simulink model "Control_test"  (R2014b)
settings: Solver=FixedStepDiscrete  StartTime=0.0  StopTime=Inf  FixedStep=0.001  RelTol=1e-3
PostLoadFcn:
  | , if any(exist('dsrtsu_mdlpostloadfcn', 'file') == [2, 3, 6]), try dsrtsu_mdlpostloadfcn('Execute', bdroot); catch fprintf('Error in PostLoadFcn (dsrtsu_mdlpostloadfcn) for model "%s":\n %s\n', bdroot, lasterr); end, end,
undefined symbols (not defined in the file or in its folder): dtLocal, slcm
libraries: rtican x163, simulink x14
(part 17 of 34)

== system Control_test/InputProcessing/RadarCanProcessing/Primary Target Selection ==
  IP : Inport
  Bus Creator : BusCreator
  Bus Selector : BusSelector  OutputSignals=ESR_Status4.CAN_TX_PATH_ID_ACC,Track01,Track02,Track03,Track04,Track05,Track06,Track07,Track08,Track09,Track10,Track11,Track12,Track13,Track14,Track15,Track16,Track17,Track18,Track19,Track20,Track21,Track22,Track23,Track24,Track25,Track26,Track27,Track28,Track29,Track30,Track31,Track32,Track33,Track34,Track35,Track36,Track37,Track38,Track39,Track40,Track41,Track42,Track43,Track44,Track45,Track46,Track47,Track48,Track49,Track50,Track51,Track52,Track53,Track54,Track55,Track56,Track57,Track58,Track59,Track60,Track61,Track62,Track63,Track64
  Default : Subsystem
  Demux : Demux  Outputs=12
  Multiport Switch1 : MultiPortSwitch  DataPortOrder=Zero-based contiguous  Inputs=65  zeroidx=on
  Terminator{,1..3,5..8} (8 alike) : Terminator
  PT : Outport
  wires:
  IP/1 -> Bus Selector/1
  Bus Selector/1 -> Multiport Switch1/1  "<CAN_TX_PATH_ID_ACC>"
  Bus Selector/2 -> Multiport Switch1/3  "<Track01>"
  Bus Selector/3 -> Multiport Switch1/4  "<Track02>"
  Bus Selector/4 -> Multiport Switch1/5  "<Track03>"
  Bus Selector/5 -> Multiport Switch1/6  "<Track04>"
  Bus Selector/6 -> Multiport Switch1/7  "<Track05>"
  Bus Selector/7 -> Multiport Switch1/8  "<Track06>"
  Bus Selector/8 -> Multiport Switch1/9  "<Track07>"
  Bus Selector/9 -> Multiport Switch1/10  "<Track08>"
  Bus Selector/10 -> Multiport Switch1/11  "<Track09>"
  Bus Selector/11 -> Multiport Switch1/12  "<Track10>"
  Bus Selector/12 -> Multiport Switch1/13  "<Track11>"
  Bus Selector/13 -> Multiport Switch1/14  "<Track12>"
  Bus Selector/14 -> Multiport Switch1/15  "<Track13>"
  Bus Selector/15 -> Multiport Switch1/16  "<Track14>"
  Bus Selector/16 -> Multiport Switch1/17  "<Track15>"
  Bus Selector/17 -> Multiport Switch1/18  "<Track16>"
  Bus Selector/18 -> Multiport Switch1/19  "<Track17>"
  Bus Selector/19 -> Multiport Switch1/20  "<Track18>"
  Bus Selector/20 -> Multiport Switch1/21  "<Track19>"
  Bus Selector/21 -> Multiport Switch1/22  "<Track20>"
  Bus Selector/22 -> Multiport Switch1/23  "<Track21>"
  Bus Selector/23 -> Multiport Switch1/24  "<Track22>"
  Bus Selector/24 -> Multiport Switch1/25  "<Track23>"
  Bus Selector/25 -> Multiport Switch1/26  "<Track24>"
  Bus Selector/26 -> Multiport Switch1/27  "<Track25>"
  Bus Selector/27 -> Multiport Switch1/28  "<Track26>"
  Bus Selector/28 -> Multiport Switch1/29  "<Track27>"
  Bus Selector/29 -> Multiport Switch1/30  "<Track28>"
  Bus Selector/30 -> Multiport Switch1/31  "<Track29>"
  Bus Selector/31 -> Multiport Switch1/32  "<Track30>"
  Bus Selector/32 -> Multiport Switch1/33  "<Track31>"
  Bus Selector/33 -> Multiport Switch1/34  "<Track32>"
  Bus Selector/34 -> Multiport Switch1/35  "<Track33>"
  Bus Selector/35 -> Multiport Switch1/36  "<Track34>"
  Bus Selector/36 -> Multiport Switch1/37  "<Track35>"
  Bus Selector/37 -> Multiport Switch1/38  "<Track36>"
  Bus Selector/38 -> Multiport Switch1/39  "<Track37>"
  Bus Selector/39 -> Multiport Switch1/40  "<Track38>"
  Bus Selector/40 -> Multiport Switch1/41  "<Track39>"
  Bus Selector/41 -> Multiport Switch1/42  "<Track40>"
  Bus Selector/42 -> Multiport Switch1/43  "<Track41>"
  Bus Selector/43 -> Multiport Switch1/44  "<Track42>"
  Bus Selector/44 -> Multiport Switch1/45  "<Track43>"
  Bus Selector/45 -> Multiport Switch1/46  "<Track44>"
  Bus Selector/46 -> Multiport Switch1/47  "<Track45>"
  Bus Selector/47 -> Multiport Switch1/48  "<Track46>"
  Bus Selector/48 -> Multiport Switch1/49  "<Track47>"
  Bus Selector/49 -> Multiport Switch1/50  "<Track48>"
  Bus Selector/50 -> Multiport Switch1/51  "<Track49>"
  Bus Selector/51 -> Multiport Switch1/52  "<Track50>"
  Bus Selector/52 -> Multiport Switch1/53  "<Track51>"
  Bus Selector/53 -> Multiport Switch1/54  "<Track52>"
  Bus Selector/54 -> Multiport Switch1/55  "<Track53>"
  Bus Selector/55 -> Multiport Switch1/56  "<Track54>"
  Bus Selector/56 -> Multiport Switch1/57  "<Track55>"
  Bus Selector/57 -> Multiport Switch1/58  "<Track56>"
  Bus Selector/58 -> Multiport Switch1/59  "<Track57>"
  Bus Selector/59 -> Multiport Switch1/60  "<Track58>"
  Bus Selector/60 -> Multiport Switch1/61  "<Track59>"
  Bus Selector/61 -> Multiport Switch1/62  "<Track60>"
  Bus Selector/62 -> Multiport Switch1/63  "<Track61>"
  Bus Selector/63 -> Multiport Switch1/64  "<Track62>"
  Bus Selector/64 -> Multiport Switch1/65  "<Track63>"
  Bus Selector/65 -> Multiport Switch1/66  "<Track64>"
  Default/1(Out1) -> Multiport Switch1/2
  Multiport Switch1/1 -> Demux/1
  Demux/1 -> Bus Creator/1  "RangeRate[m/s]"
  Demux/3 -> Bus Creator/2  "RangeAccel[m/s2]"
  Demux/7 -> Bus Creator/3  "Range[m]"
  Bus Creator/1 -> PT/1  "PT_Data"
  Demux/2 -> Terminator/1
  Demux/4 -> Terminator1/1
  Demux/5 -> Terminator2/1
  Demux/6 -> Terminator3/1
  Demux/9 -> Terminator5/1
  Demux/10 -> Terminator6/1
  Demux/11 -> Terminator7/1
  Demux/12 -> Terminator8/1
  Demux/8 -> Bus Creator/4  "Angle[deg]"

== system Control_test/InputProcessing/RadarCanProcessing/Status4 ==
  Bus Creator : BusCreator  Inputs=13
  Bus Selector : BusSelector  OutputSignals=CAN_TX_PATH_ID_ACC
  ESR_Status4 : rtican/RTICAN Receive (RX)   Reserved1=[]  Reserved2=[]  Reserved3=[]  Reserved4=[]  SfcnMessage=[]  Msg_Struct=[]  BoardTypeNo=[]  BoardNo=[]  ChannelNo=[]  Parameters=[]  DialogFcn=[]  UnitName=[]  Revision=[]  UnitValues=[]  DSProperties=struct('RTI',struct('Version',uint32(5),'BlockType',struct('isSLSource',uint8(1),'isSLSink',uint8(1),'isHWSource',uint8(0),'isHWSink',uint8(0),'isSetup',uint8(0),'isInline',uint8(1),'isNonInline',uint8(0),'isInterrupt',uint8(0),'isChannelwise',uint8(0)),'IOBoardType','RTICAN','UnitType','MESSAGE','Identifier','RX','DialogType','MSVC','BlockSet','RTICAN','SlaveProcessor','CAN'))  RTIBlockInterface=struct('OutputPortsWidth',int32([1 1 1 1 1 1 1 1 1 1 1 1 1]),'OutputPortsActive',[1 1 1 1 1 1 1 1 1 1 1 1 1],'OutputPortsName',{{'CAN_TX_PATH_ID_ACC_STAT','CAN_TX_AUTO_ALIGN_ANGLE','CAN_TX_PATH_ID_FCW_STAT','CAN_TX_PATH_ID_FCW_MOVE','CAN_TX_PATH_ID_CMBB_STAT','CAN_TX_PATH_ID_CMBB_MOVE','CAN_TX_PATH_ID_ACC','CAN_TX_ROLLING_COUNT_3','CAN_TX_MR_LR_MODE','CAN_TX_PARTIAL_BLOCKAGE','CAN_TX_SIDELOBE_BLOCKAGE','CAN_TX_LR_ONLY_GRATING_LOBE_DET','CAN_TX_TRUCK_TARGET_DET'}},'OutputPortsDataType',{{'SS_DOUBLE','SS_DOUBLE','SS_DOUBLE','SS_DOUBLE','SS_DOUBLE','SS_DOUBLE','SS_DOUBLE','SS_DOUBLE','SS_DOUBLE','SS_DOUBLE','SS_DOUBLE','SS_DOUBLE','SS_DOUBLE'}},'OutputPortsLabel',{{'CAN_TX_PATH_ID_ACC_STAT','CAN_TX_AUTO_ALIGN_ANGLE','CAN_TX_PATH_ID_FCW_STAT','CAN_TX_PATH_ID_FCW_MOVE','CAN_TX_PATH_ID_CMBB_STAT','CAN_TX_PATH_ID_CMBB_MOVE','CAN_TX_PATH_ID_ACC','CAN_TX_ROLLING_COUNT_3','CAN_TX_MR_LR_MODE','CAN_TX_PARTIAL_BLOCKAGE','CAN_TX_SIDELOBE_BLOCKAGE','CAN_TX_LR_ONLY_GRATING_LOBE_DET','CAN_TX_TRUCK_TARGET_DET'}},'OutputPortsLabelMode','ON','InputPortsWidth',int32(0),'InputPortsActive',0,'DialogFcn','rtican_message_interface_gui','BlockDisplay',{{'','center'}},'IconTransparency','on','ParameterTunableNames',{{}},'InitLevel',3,'BlockName',struct('Token',{{'ESR_Status4'}}),'SampleTime',{{0.01}},'TriggerPort',{{'none'}},'EnablePort',{{'none'}})  RTIBlockParameters=struct('BoardTypeNo',{{1,'OFF',[]}},'BoardNo',{{2,'ON',[1 16]}},'ChannelNo',{{2,'ON',[1 2]}},'Parameters',{{struct('DataFileSupport',struct('DataFileSelectedMaster',1,'DataFileSelectedLocal',0,'DataFileName','c:\users\mpc_car\documents\github\mpc-car\dbcfiles\esr_dv3_64tgt.dbc|','DataFileDate',{{{['26-Aug-2014 13:16:21']}}},'SelectedFile',['<no file selected>'],'InterfaceFcn','rtican_dbc_file_parser'),'Options',struct('StatusSelected',0,'TimeSelected',0,'DeltaTimeSelected',0,'BytePortSelected',0,'MessageLengthSelected',0,'TriggerPort',struct('Selected',0,'TriggerType',0),'UserCoding',struct('Selected',0,'InterfaceFile','UserDecodingFile','FcnName','UserDecodeFcn','InportSelected',0,'InportWidth',1,'OutportSelected',0,'OutportWidth',1),'EnablePortSelected',0,'SignalOnPortnameSelected',1,'UseRXService',0),'Message',struct('MsgOnBlocknameSelected',1,'MsgName','ESR_Status4','MsgIdFormat',0,'MsgId',1251,'MsgLength',8,'NumSignals',13,'SampleTime',0.01,'Signal',struct('SgnName',{'CAN_TX_PATH_ID_ACC_STAT','CAN_TX_AUTO_ALIGN_ANGLE','CAN_TX_PATH_ID_FCW_STAT','CAN_TX_PATH_ID_FCW_MOVE','CAN_TX_PATH_ID_CMBB_STAT','CAN_TX_PATH_ID_CMBB_MOVE','CAN_TX_PATH_ID_ACC','CAN_TX_ROLLING_COUNT_3','CAN_TX_MR_LR_MODE','CAN_TX_PARTIAL_BLOCKAGE','CAN_TX_SIDELOBE_BLOCKAGE','CAN_TX_LR_ONLY_GRATING_LOBE_DET','CAN_TX_TRUCK_TARGET_DET'},'SgnStartBit',{0,8,16,24,32,40,48,56,58,60,61,62,63},'SgnLength',{8,8,8,8,8,8,8,2,2,1,1,1,1},'SgnType',{0,0,0,0,0,0,0,0,0,0,0,0,0},'ModeValue',{-1,-1,-1,-1,-1,-1,-1,-1,-1,-1,-1,-1,-1},'DataType',{0,1,0,0,0,0,0,0,0,0,0,0,0},'ByteLayout',{2,2,2,2,2,2,2,2,2,2,2,2,2},'Factor',{1,0.0625,1,1,1,1,1,1,1,1,1,1,1},'Offset',{0,0,0,0,0,0,0,0,0,0,0,0,0},'SgnComment',{{''},{''},{''},{''},{''},{''},{''},{''},{''},{''},{''},{''},{''}},'SgnUnit',{'','','','','','','','','','','','',''},'Min',{0,-8,0,0,0,0,0,0,0,0,0,0,0},'Max',{0,7.9375,0,0,0,0,0,0,3,0,0,0,0},'SLDataType',{'SS_DOUBLE','SS_DOUBLE','SS_DOUBLE','SS_DOUBLE','SS_DOUBLE','SS_DOUBLE','SS_DOUBLE','SS_DOUBLE','SS_DOUBLE','SS_DOUBLE','SS_DOUBLE','SS_DOUBLE','SS_DOUBLE'}),'MsgIdNumFormat',0,'MsgComment',{{''}}),'Version',1.2,'general',struct('isFromLib',0)),'OFF',[]}},'GroupId',{{struct('Group',{{'RTICAN'}},'No',4,'Behavior',{{'NAMECHANGE'}},'BlockType',{{'SINK'}},'NameChangeFlag',0),'OFF',[]}},'SFcnRTICANMessage',{{struct('MsgType','RX','SFcnPortType','Scalar','MsgName','ESR_Status4','MsgIdFormat','STD','MsgId',1251,'MsgLength',8,'NumSignals',13,'SampleTime',0.01,'Signal',struct('SgnName',{'CAN_TX_PATH_ID_ACC_STAT','CAN_TX_AUTO_ALIGN_ANGLE','CAN_TX_PATH_ID_FCW_STAT','CAN_TX_PATH_ID_FCW_MOVE','CAN_TX_PATH_ID_CMBB_STAT','CAN_TX_PATH_ID_CMBB_MOVE','CAN_TX_PATH_ID_ACC','CAN_TX_ROLLING_COUNT_3','CAN_TX_MR_LR_MODE','CAN_TX_PARTIAL_BLOCKAGE','CAN_TX_SIDELOBE_BLOCKAGE','CAN_TX_LR_ONLY_GRATING_LOBE_DET','CAN_TX_TRUCK_TARGET_DET'},'SgnStartBit',{0,8,16,24,32,40,48,56,58,60,61,62,63},'SgnLength',{8,8,8,8,8,8,8,2,2,1,1,1,1},'SgnType',{'standard','standard','standard','standard','standard','standard','standard','standard','standard','standard','standard','standard','standard'},'ModeValue',{-1,-1,-1,-1,-1,-1,-1,-1,-1,-1,-1,-1,-1},'DataType',{['unsigned int'],['signed int'],['unsigned int'],['unsigned int'],['unsigned int'],['unsigned int'],['unsigned int'],['unsigned int'],['unsigned int'],['unsigned int'],['unsigned int'],['unsigned int'],['unsigned int']},'ByteLayout',{['motorola back.'],['motorola back.'],['motorola back.'],['motorola back.'],['motorola back.'],['motorola back.'],['motorola back.'],['motorola back.'],['motorola back.'],['motorola back.'],['motorola back.'],['motorola back.'],['motorola back.']},'Factor',{1,0.0625,1,1,1,1,1,1,1,1,1,1,1},'Offset',{0,0,0,0,0,0,0,0,0,0,0,0,0},'SLDataType',{'SS_DOUBLE','SS_DOUBLE','SS_DOUBLE','SS_DOUBLE','SS_DOUBLE','SS_DOUBLE','SS_DOUBLE','SS_DOUBLE','SS_DOUBLE','SS_DOUBLE','SS_DOUBLE','SS_DOUBLE','SS_DOUBLE'}),'StatusSelected','no','TimeSelected','no','DeltaTimeSelected','no','BytePortSelected','no','MessageLengthSelected','no','TriggerPort',struct('Selected','no','TriggerType',0),'UserCoding',struct('Selected','no','InterfaceFile','UserDecodingFile','FcnName','UserDecodeFcn','InportSelected','no','InportWidth',1,'OutportSelected','no','OutportWidth',1),'EnablePortSelected','no','UseRXService','no','BoardType','DS1','BoardNo',2,'ControllerNo',2),'OFF',[]}},'TLCFileName',{{'rtican_rx_message','OFF',[]}})  RTISFcnParameters=struct('SFcnRTICANMessage','struct','TLCFileName','char')  RTIBlockParaDefault=struct('BoardTypeNo',4302,'BoardNo',1,'ChannelNo',1,'Parameters',struct('DataFileSupport',struct('DataFileSelectedMaster',0,'DataFileSelectedLocal',0,'DataFileName','','DataFileDate','','SelectedFile',['<no file selected>']),'Options',struct('StatusSelected',1,'TimeSelected',1,'DeltaTimeSelected',1,'BytePortSelected',0,'MessageLengthSelected',0,'TriggerPort',struct('Selected',0,'TriggerType','rising'),'UserCoding',struct('Selected',0,'InterfaceFile','UserDecodingFile','FcnName','UserDecodeFcn','InportSelected',0,'InportWidth',1,'OutportSelected',0,'OutportWidth',1),'EnablePortSelected',0,'SignalOnPortnameSelected',1,'UseRXService',0),'Message',struct('MsgOnBlocknameSelected',0,'MsgName',['RX Message'],'MsgIdFormat',0,'MsgId',100,'MsgLength',8,'NumSignals',1,'SampleTime',-1,'Signal',struct('SgnName',['RX signal'],'SgnStartBit',0,'SgnLength',8,'SgnType',0,'ModeValue',-1,'DataType',0,'SLDataType','SS_DOUBLE','ByteLayout',0,'Factor',1,'Offset',0,'Min',0,'Max',255,'SgnComment',{{}},'SgnUnit',''),'MsgIdNumFormat',0,'MsgComment',{{''}}),'Version',1.2,'general',struct('isFromLib',1)),'GroupId',struct('Group',{{'RTICAN'}},'No',1,'Behavior',{{'NAMECHANGE'}},'BlockType',{{'SINK'}},'NameChangeFlag',0),'SFcnRTICANMessage',struct('MsgType','RX','MsgName',['RX Message'],'MsgIdFormat','STD','MsgId',100,'MsgLength',8,'NumSignals',1,'SampleTime',-1,'Signal',struct('SgnName',['RX signal'],'SgnStartBit',0,'SgnLength',8,'SgnType','standard','ModeValue',-1,'DataType',['unsigned int'],'ByteLayout',['little endian'],'SLDataType','SS_DOUBLE','Factor',1,'Offset',0),'StatusSelected','yes','TimeSelected','yes','DeltaTimeSelected','yes','BytePortSelected','no','MessageLengthSelected','no','EnablePortSelected','no','UserCoding',struct('Selected','no','InterfaceFile','UserDecodingFile','FcnName','UserDecodeFcn','InportSelected','no','InportWidth',1,'OutportSelected','no','OutportWidth',1),'TriggerPort',struct('Selected','no','TriggerType','rising'),'UseRXService','no','BoardType','DS4302','BoardNo',1,'ControllerNo',1,'SFcnPortType','Scalar'),'TLCFileName','rtican_rx_message')
      settings: AttributesFormatString=Group Id: RTICAN4\n
  CAN_TX_PATH_ID_ACC : Outport
  wires:
  ESR_Status4/1 -> Bus Creator/1  "CAN_TX_PATH_ID_ACC_STAT"
  ESR_Status4/2 -> Bus Creator/2  "CAN_TX_AUTO_ALIGN_ANGLE"
  ESR_Status4/3 -> Bus Creator/3  "CAN_TX_PATH_ID_FCW_STAT"
  ESR_Status4/4 -> Bus Creator/4  "CAN_TX_PATH_ID_FCW_MOVE"
  ESR_Status4/5 -> Bus Creator/5  "CAN_TX_PATH_ID_CMBB_STAT"
  ESR_Status4/6 -> Bus Creator/6  "CAN_TX_PATH_ID_CMBB_MOVE"
  ESR_Status4/7 -> Bus Creator/7  "CAN_TX_PATH_ID_ACC"
  ESR_Status4/8 -> Bus Creator/8  "CAN_TX_ROLLING_COUNT_3"
  ESR_Status4/9 -> Bus Creator/9  "CAN_TX_MR_LR_MODE"
  ESR_Status4/10 -> Bus Creator/10  "CAN_TX_PARTIAL_BLOCKAGE"
  ESR_Status4/11 -> Bus Creator/11  "CAN_TX_SIDELOBE_BLOCKAGE"
  ESR_Status4/12 -> Bus Creator/12  "CAN_TX_LR_ONLY_GRATING_LOBE_DET"
  ESR_Status4/13 -> Bus Creator/13  "CAN_TX_TRUCK_TARGET_DET"
  Bus Creator/1 -> Bus Selector/1  "Status4"
  Bus Selector/1 -> CAN_TX_PATH_ID_ACC/1  "<CAN_TX_PATH_ID_ACC>"

== system Control_test/InputProcessing/RadarCanProcessing/Track01 ==
  Bus Creator : BusCreator  Inputs=12
  ESR_Track01 : rtican/RTICAN Receive (RX)   Reserved1=[]  Reserved2=[]  Reserved3=[]  Reserved4=[]  SfcnMessage=[]  Msg_Struct=[]  BoardTypeNo=[]  BoardNo=[]  ChannelNo=[]  Parameters=[]  DialogFcn=[]  UnitName=[]  Revision=[]  UnitValues=[]  DSProperties=struct('RTI',struct('Version',uint32(5),'BlockType',struct('isSLSource',uint8(1),'isSLSink',uint8(1),'isHWSource',uint8(0),'isHWSink',uint8(0),'isSetup',uint8(0),'isInline',uint8(1),'isNonInline',uint8(0),'isInterrupt',uint8(0),'isChannelwise',uint8(0)),'IOBoardType','RTICAN','UnitType','MESSAGE','Identifier','RX','DialogType','MSVC','BlockSet','RTICAN','SlaveProcessor','CAN'))  RTIBlockInterface=struct('OutputPortsWidth',int32([1 1 1 1 1 1 1 1 1 1 1 1]),'OutputPortsActive',[1 1 1 1 1 1 1 1 1 1 1 1],'OutputPortsName',{{'CAN_TX_TRACK_RANGE_RATE_01','CAN_TX_TRACK_MED_RANGE_MODE_01','CAN_TX_TRACK_RANGE_ACCEL_01','CAN_TX_TRACK_WIDTH_01','CAN_TX_TRACK_ROLLING_COUNT_01','CAN_TX_TRACK_BRIDGE_OBJECT_01','CAN_TX_TRACK_RANGE_01','CAN_TX_TRACK_ANGLE_01','CAN_TX_TRACK_STATUS_01','CAN_TX_TRACK_ONCOMING_01','CAN_TX_TRACK_GROUPING_CHANGED_01','CAN_TX_TRACK_LAT_RATE_01'}},'OutputPortsDataType',{{'SS_DOUBLE','SS_DOUBLE','SS_DOUBLE','SS_DOUBLE','SS_DOUBLE','SS_DOUBLE','SS_DOUBLE','SS_DOUBLE','SS_DOUBLE','SS_DOUBLE','SS_DOUBLE','SS_DOUBLE'}},'OutputPortsLabel',{{'CAN_TX_TRACK_RANGE_RATE_01','CAN_TX_TRACK_MED_RANGE_MODE_01','CAN_TX_TRACK_RANGE_ACCEL_01','CAN_TX_TRACK_WIDTH_01','CAN_TX_TRACK_ROLLING_COUNT_01','CAN_TX_TRACK_BRIDGE_OBJECT_01','CAN_TX_TRACK_RANGE_01','CAN_TX_TRACK_ANGLE_01','CAN_TX_TRACK_STATUS_01','CAN_TX_TRACK_ONCOMING_01','CAN_TX_TRACK_GROUPING_CHANGED_01','CAN_TX_TRACK_LAT_RATE_01'}},'OutputPortsLabelMode','ON','InputPortsWidth',int32(0),'InputPortsActive',0,'DialogFcn','rtican_message_interface_gui','BlockDisplay',{{'','center'}},'IconTransparency','on','ParameterTunableNames',{{}},'InitLevel',3,'BlockName',struct('Token',{{'ESR_Track01'}}),'SampleTime',{{0.01}},'TriggerPort',{{'none'}},'EnablePort',{{'none'}})  RTIBlockParameters=struct('BoardTypeNo',{{1,'OFF',[]}},'BoardNo',{{2,'ON',[1 16]}},'ChannelNo',{{2,'ON',[1 2]}},'Parameters',{{struct('DataFileSupport',struct('DataFileSelectedMaster',1,'DataFileSelectedLocal',1,'DataFileName','c:\users\mpc_car\documents\github\mpc-car\controller\dbcfiles\esr_dv3_64tgt.dbc|','DataFileDate',['26-Aug-2014 13:16:21'],'SelectedFile','..\..\dbcfiles\esr_dv3_64tgt.dbc','InterfaceFcn','rtican_dbc_file_parser'),'Options',struct('StatusSelected',0,'TimeSelected',0,'DeltaTimeSelected',0,'BytePortSelected',0,'MessageLengthSelected',0,'TriggerPort',struct('Selected',0,'TriggerType',0),'UserCoding',struct('Selected',0,'InterfaceFile','UserDecodingFile','FcnName','UserDecodeFcn','InportSelected',0,'InportWidth',1,'OutportSelected',0,'OutportWidth',1),'EnablePortSelected',0,'SignalOnPortnameSelected',1,'UseRXService',0),'Message',struct('MsgOnBlocknameSelected',1,'MsgName','ESR_Track01','MsgIdFormat',0,'MsgId',1280,'MsgLength',8,'NumSignals',12,'SampleTime',0.01,'Signal',struct('SgnName',{'CAN_TX_TRACK_RANGE_RATE_01','CAN_TX_TRACK_MED_RANGE_MODE_01','CAN_TX_TRACK_RANGE_ACCEL_01','CAN_TX_TRACK_WIDTH_01','CAN_TX_TRACK_ROLLING_COUNT_01','CAN_TX_TRACK_BRIDGE_OBJECT_01','CAN_TX_TRACK_RANGE_01','CAN_TX_TRACK_ANGLE_01','CAN_TX_TRACK_STATUS_01','CAN_TX_TRACK_ONCOMING_01','CAN_TX_TRACK_GROUPING_CHANGED_01','CAN_TX_TRACK_LAT_RATE_01'},'SgnStartBit',{0,14,16,26,30,31,32,43,53,56,57,58},'SgnLength',{14,2,10,4,1,1,11,10,3,1,1,6},'ByteLayout',{2,2,2,2,2,2,2,2,2,2,2,2},'Factor',{0.01,1,0.05,0.5,1,1,0.1,0.1,1,1,1,0.25},'Offset',{0,0,0,0,0,0,0,0,0,0,0,0},'SgnComment',{'','','','','','','','','','','',''},'SgnUnit',{'m/s','','m/s/s','m','','','m','deg','','','',''},'Min',{-81.92,0,-25.6,0,0,0,0,-51.2,0,0,0,-8},'Max',{81.91,3,25.55,7.5,1,0,204.7,51.1,7,0,0,7.75},'SgnType',{0,0,0,0,0,0,0,0,0,0,0,0},'SLDataType',{'SS_DOUBLE','SS_DOUBLE','SS_DOUBLE','SS_DOUBLE','SS_DOUBLE','SS_DOUBLE','SS_DOUBLE','SS_DOUBLE','SS_DOUBLE','SS_DOUBLE','SS_DOUBLE','SS_DOUBLE'},'DataType',{1,0,1,0,0,0,0,1,0,0,0,1},'ModeValue',{-1,-1,-1,-1,-1,-1,-1,-1,-1,-1,-1,-1}),'MsgIdNumFormat',0,'MsgComment',{{''}}),'Version',1.2,'general',struct('isFromLib',0)),'OFF',[]}},'GroupId',{{struct('Group',{{'RTICAN'}},'No',4,'Behavior',{{'NAMECHANGE'}},'BlockType',{{'SINK'}},'NameChangeFlag',0),'OFF',[]}},'SFcnRTICANMessage',{{struct('MsgType','RX','SFcnPortType','Scalar','MsgName','ESR_Track01','MsgIdFormat','STD','MsgId',1280,'MsgLength',8,'NumSignals',12,'SampleTime',0.01,'Signal',struct('SgnName',{'CAN_TX_TRACK_RANGE_RATE_01','CAN_TX_TRACK_MED_RANGE_MODE_01','CAN_TX_TRACK_RANGE_ACCEL_01','CAN_TX_TRACK_WIDTH_01','CAN_TX_TRACK_ROLLING_COUNT_01','CAN_TX_TRACK_BRIDGE_OBJECT_01','CAN_TX_TRACK_RANGE_01','CAN_TX_TRACK_ANGLE_01','CAN_TX_TRACK_STATUS_01','CAN_TX_TRACK_ONCOMING_01','CAN_TX_TRACK_GROUPING_CHANGED_01','CAN_TX_TRACK_LAT_RATE_01'},'SgnStartBit',{0,14,16,26,30,31,32,43,53,56,57,58},'SgnLength',{14,2,10,4,1,1,11,10,3,1,1,6},'ByteLayout',{['motorola back.'],['motorola back.'],['motorola back.'],['motorola back.'],['motorola back.'],['motorola back.'],['motorola back.'],['motorola back.'],['motorola back.'],['motorola back.'],['motorola back.'],['motorola back.']},'Factor',{0.01,1,0.05,0.5,1,1,0.1,0.1,1,1,1,0.25},'Offset',{0,0,0,0,0,0,0,0,0,0,0,0},'SgnType',{'standard','standard','standard','standard','standard','standard','standard','standard','standard','standard','standard','standard'},'SLDataType',{'SS_DOUBLE','SS_DOUBLE','SS_DOUBLE','SS_DOUBLE','SS_DOUBLE','SS_DOUBLE','SS_DOUBLE','SS_DOUBLE','SS_DOUBLE','SS_DOUBLE','SS_DOUBLE','SS_DOUBLE'},'DataType',{['signed int'],['unsigned int'],['signed int'],['unsigned int'],['unsigned int'],['unsigned int'],['unsigned int'],['signed int'],['unsigned int'],['unsigned int'],['unsigned int'],['signed int']},'ModeValue',{-1,-1,-1,-1,-1,-1,-1,-1,-1,-1,-1,-1}),'StatusSelected','no','TimeSelected','no','DeltaTimeSelected','no','BytePortSelected','no','MessageLengthSelected','no','TriggerPort',struct('Selected','no','TriggerType',0),'UserCoding',struct('Selected','no','InterfaceFile','UserDecodingFile','FcnName','UserDecodeFcn','InportSelected','no','InportWidth',1,'OutportSelected','no','OutportWidth',1),'EnablePortSelected','no','UseRXService','no','BoardType','DS1','BoardNo',2,'ControllerNo',2),'OFF',[]}},'TLCFileName',{{'rtican_rx_message','OFF',[]}})  RTISFcnParameters=struct('SFcnRTICANMessage','struct','TLCFileName','char')  RTIBlockParaDefault=struct('BoardTypeNo',4302,'BoardNo',1,'ChannelNo',1,'Parameters',struct('DataFileSupport',struct('DataFileSelectedMaster',0,'DataFileSelectedLocal',0,'DataFileName','','DataFileDate','','SelectedFile',['<no file selected>']),'Options',struct('StatusSelected',1,'TimeSelected',1,'DeltaTimeSelected',1,'BytePortSelected',0,'MessageLengthSelected',0,'TriggerPort',struct('Selected',0,'TriggerType','rising'),'UserCoding',struct('Selected',0,'InterfaceFile','UserDecodingFile','FcnName','UserDecodeFcn','InportSelected',0,'InportWidth',1,'OutportSelected',0,'OutportWidth',1),'EnablePortSelected',0,'SignalOnPortnameSelected',1,'UseRXService',0),'Message',struct('MsgOnBlocknameSelected',0,'MsgName',['RX Message'],'MsgIdFormat',0,'MsgId',100,'MsgLength',8,'NumSignals',1,'SampleTime',-1,'Signal',struct('SgnName',['RX signal'],'SgnStartBit',0,'SgnLength',8,'SgnType',0,'ModeValue',-1,'DataType',0,'SLDataType','SS_DOUBLE','ByteLayout',0,'Factor',1,'Offset',0,'Min',0,'Max',255,'SgnComment',{{}},'SgnUnit',''),'MsgIdNumFormat',0,'MsgComment',{{''}}),'Version',1.2,'general',struct('isFromLib',1)),'GroupId',struct('Group',{{'RTICAN'}},'No',1,'Behavior',{{'NAMECHANGE'}},'BlockType',{{'SINK'}},'NameChangeFlag',0),'SFcnRTICANMessage',struct('MsgType','RX','MsgName',['RX Message'],'MsgIdFormat','STD','MsgId',100,'MsgLength',8,'NumSignals',1,'SampleTime',-1,'Signal',struct('SgnName',['RX signal'],'SgnStartBit',0,'SgnLength',8,'SgnType','standard','ModeValue',-1,'DataType',['unsigned int'],'ByteLayout',['little endian'],'SLDataType','SS_DOUBLE','Factor',1,'Offset',0),'StatusSelected','yes','TimeSelected','yes','DeltaTimeSelected','yes','BytePortSelected','no','MessageLengthSelected','no','EnablePortSelected','no','UserCoding',struct('Selected','no','InterfaceFile','UserDecodingFile','FcnName','UserDecodeFcn','InportSelected','no','InportWidth',1,'OutportSelected','no','OutportWidth',1),'TriggerPort',struct('Selected','no','TriggerType','rising'),'UseRXService','no','BoardType','DS4302','BoardNo',1,'ControllerNo',1,'SFcnPortType','Scalar'),'TLCFileName','rtican_rx_message')
      settings: AttributesFormatString=Group Id: RTICAN4\n
  Out1 : Outport
  wires:
  ESR_Track01/1 -> Bus Creator/1  "CAN_TX_TRACK_RANGE_RATE_01"
  ESR_Track01/2 -> Bus Creator/2  "CAN_TX_TRACK_MED_RANGE_MODE_01"
  ESR_Track01/3 -> Bus Creator/3  "CAN_TX_TRACK_RANGE_ACCEL_01"
  ESR_Track01/4 -> Bus Creator/4  "CAN_TX_TRACK_WIDTH_01"
  ESR_Track01/5 -> Bus Creator/5  "CAN_TX_TRACK_ROLLING_COUNT_01"
  ESR_Track01/6 -> Bus Creator/6  "CAN_TX_TRACK_BRIDGE_OBJECT_01"
  ESR_Track01/7 -> Bus Creator/7  "CAN_TX_TRACK_RANGE_01"
  ESR_Track01/8 -> Bus Creator/8  "CAN_TX_TRACK_ANGLE_01"
  ESR_Track01/9 -> Bus Creator/9  "CAN_TX_TRACK_STATUS_01"
  ESR_Track01/10 -> Bus Creator/10  "CAN_TX_TRACK_ONCOMING_01"
  ESR_Track01/11 -> Bus Creator/11  "CAN_TX_TRACK_GROUPING_CHANGED_01"
  ESR_Track01/12 -> Bus Creator/12  "CAN_TX_TRACK_LAT_RATE_01"
  Bus Creator/1 -> Out1/1  "Track01"

== system Control_test/InputProcessing/RadarCanProcessing/Track02 ==
  Bus Creator : BusCreator  Inputs=12
  ESR_Track02 : rtican/RTICAN Receive (RX)   Reserved1=[]  Reserved2=[]  Reserved3=[]  Reserved4=[]  SfcnMessage=[]  Msg_Struct=[]  BoardTypeNo=[]  BoardNo=[]  ChannelNo=[]  Parameters=[]  DialogFcn=[]  UnitName=[]  Revision=[]  UnitValues=[]  DSProperties=struct('RTI',struct('Version',uint32(5),'BlockType',struct('isSLSource',uint8(1),'isSLSink',uint8(1),'isHWSource',uint8(0),'isHWSink',uint8(0),'isSetup',uint8(0),'isInline',uint8(1),'isNonInline',uint8(0),'isInterrupt',uint8(0),'isChannelwise',uint8(0)),'IOBoardType','RTICAN','UnitType','MESSAGE','Identifier','RX','DialogType','MSVC','BlockSet','RTICAN','SlaveProcessor','CAN'))  RTIBlockInterface=struct('OutputPortsWidth',int32([1 1 1 1 1 1 1 1 1 1 1 1]),'OutputPortsActive',[1 1 1 1 1 1 1 1 1 1 1 1],'OutputPortsName',{{'CAN_TX_TRACK_RANGE_RATE_02','CAN_TX_TRACK_MED_RANGE_MODE_02','CAN_TX_TRACK_RANGE_ACCEL_02','CAN_TX_TRACK_WIDTH_02','CAN_TX_TRACK_ROLLING_COUNT_02','CAN_TX_TRACK_BRIDGE_OBJECT_02','CAN_TX_TRACK_RANGE_02','CAN_TX_TRACK_ANGLE_02','CAN_TX_TRACK_STATUS_02','CAN_TX_TRACK_ONCOMING_02','CAN_TX_TRACK_GROUPING_CHANGED_02','CAN_TX_TRACK_LAT_RATE_02'}},'OutputPortsDataType',{{'SS_DOUBLE','SS_DOUBLE','SS_DOUBLE','SS_DOUBLE','SS_DOUBLE','SS_DOUBLE','SS_DOUBLE','SS_DOUBLE','SS_DOUBLE','SS_DOUBLE','SS_DOUBLE','SS_DOUBLE'}},'OutputPortsLabel',{{'CAN_TX_TRACK_RANGE_RATE_02','CAN_TX_TRACK_MED_RANGE_MODE_02','CAN_TX_TRACK_RANGE_ACCEL_02','CAN_TX_TRACK_WIDTH_02','CAN_TX_TRACK_ROLLING_COUNT_02','CAN_TX_TRACK_BRIDGE_OBJECT_02','CAN_TX_TRACK_RANGE_02','CAN_TX_TRACK_ANGLE_02','CAN_TX_TRACK_STATUS_02','CAN_TX_TRACK_ONCOMING_02','CAN_TX_TRACK_GROUPING_CHANGED_02','CAN_TX_TRACK_LAT_RATE_02'}},'OutputPortsLabelMode','ON','InputPortsWidth',int32(0),'InputPortsActive',0,'DialogFcn','rtican_message_interface_gui','BlockDisplay',{{'','center'}},'IconTransparency','on','ParameterTunableNames',{{}},'InitLevel',3,'BlockName',struct('Token',{{'ESR_Track02'}}),'SampleTime',{{0.01}},'TriggerPort',{{'none'}},'EnablePort',{{'none'}})  RTIBlockParameters=struct('BoardTypeNo',{{1,'OFF',[]}},'BoardNo',{{2,'ON',[1 16]}},'ChannelNo',{{2,'ON',[1 2]}},'Parameters',{{struct('DataFileSupport',struct('DataFileSelectedMaster',1,'DataFileSelectedLocal',1,'DataFileName','c:\users\mpc_car\documents\github\mpc-car\controller\dbcfiles\esr_dv3_64tgt.dbc|','DataFileDate',['26-Aug-2014 13:16:21'],'SelectedFile','..\..\dbcfiles\esr_dv3_64tgt.dbc','InterfaceFcn','rtican_dbc_file_parser'),'Options',struct('StatusSelected',0,'TimeSelected',0,'DeltaTimeSelected',0,'BytePortSelected',0,'MessageLengthSelected',0,'TriggerPort',struct('Selected',0,'TriggerType',0),'UserCoding',struct('Selected',0,'InterfaceFile','UserDecodingFile','FcnName','UserDecodeFcn','InportSelected',0,'InportWidth',1,'OutportSelected',0,'OutportWidth',1),'EnablePortSelected',0,'SignalOnPortnameSelected',1,'UseRXService',0),'Message',struct('MsgOnBlocknameSelected',1,'MsgName','ESR_Track02','MsgIdFormat',0,'MsgId',1281,'MsgLength',8,'NumSignals',12,'SampleTime',0.01,'Signal',struct('SgnName',{'CAN_TX_TRACK_RANGE_RATE_02','CAN_TX_TRACK_MED_RANGE_MODE_02','CAN_TX_TRACK_RANGE_ACCEL_02','CAN_TX_TRACK_WIDTH_02','CAN_TX_TRACK_ROLLING_COUNT_02','CAN_TX_TRACK_BRIDGE_OBJECT_02','CAN_TX_TRACK_RANGE_02','CAN_TX_TRACK_ANGLE_02','CAN_TX_TRACK_STATUS_02','CAN_TX_TRACK_ONCOMING_02','CAN_TX_TRACK_GROUPING_CHANGED_02','CAN_TX_TRACK_LAT_RATE_02'},'SgnStartBit',{0,14,16,26,30,31,32,43,53,56,57,58},'SgnLength',{14,2,10,4,1,1,11,10,3,1,1,6},'ByteLayout',{2,2,2,2,2,2,2,2,2,2,2,2},'Factor',{0.01,1,0.05,0.5,1,1,0.1,0.1,1,1,1,0.25},'Offset',{0,0,0,0,0,0,0,0,0,0,0,0},'SgnComment',{'','','','','','','','','','','',''},'SgnUnit',{'m/s','','m/s/s','m','','','m','deg','','','',''},'Min',{-81.92,0,-25.6,0,0,0,0,-51.2,0,0,0,-8},'Max',{81.91,3,25.55,7.5,1,0,204.7,51.1,7,0,0,7.75},'SgnType',{0,0,0,0,0,0,0,0,0,0,0,0},'SLDataType',{'SS_DOUBLE','SS_DOUBLE','SS_DOUBLE','SS_DOUBLE','SS_DOUBLE','SS_DOUBLE','SS_DOUBLE','SS_DOUBLE','SS_DOUBLE','SS_DOUBLE','SS_DOUBLE','SS_DOUBLE'},'DataType',{1,0,1,0,0,0,0,1,0,0,0,1},'ModeValue',{-1,-1,-1,-1,-1,-1,-1,-1,-1,-1,-1,-1}),'MsgIdNumFormat',0,'MsgComment',{{''}}),'Version',1.2,'general',struct('isFromLib',0)),'OFF',[]}},'GroupId',{{struct('Group',{{'RTICAN'}},'No',4,'Behavior',{{'NAMECHANGE'}},'BlockType',{{'SINK'}},'NameChangeFlag',0),'OFF',[]}},'SFcnRTICANMessage',{{struct('MsgType','RX','SFcnPortType','Scalar','MsgName','ESR_Track02','MsgIdFormat','STD','MsgId',1281,'MsgLength',8,'NumSignals',12,'SampleTime',0.01,'Signal',struct('SgnName',{'CAN_TX_TRACK_RANGE_RATE_02','CAN_TX_TRACK_MED_RANGE_MODE_02','CAN_TX_TRACK_RANGE_ACCEL_02','CAN_TX_TRACK_WIDTH_02','CAN_TX_TRACK_ROLLING_COUNT_02','CAN_TX_TRACK_BRIDGE_OBJECT_02','CAN_TX_TRACK_RANGE_02','CAN_TX_TRACK_ANGLE_02','CAN_TX_TRACK_STATUS_02','CAN_TX_TRACK_ONCOMING_02','CAN_TX_TRACK_GROUPING_CHANGED_02','CAN_TX_TRACK_LAT_RATE_02'},'SgnStartBit',{0,14,16,26,30,31,32,43,53,56,57,58},'SgnLength',{14,2,10,4,1,1,11,10,3,1,1,6},'ByteLayout',{['motorola back.'],['motorola back.'],['motorola back.'],['motorola back.'],['motorola back.'],['motorola back.'],['motorola back.'],['motorola back.'],['motorola back.'],['motorola back.'],['motorola back.'],['motorola back.']},'Factor',{0.01,1,0.05,0.5,1,1,0.1,0.1,1,1,1,0.25},'Offset',{0,0,0,0,0,0,0,0,0,0,0,0},'SgnType',{'standard','standard','standard','standard','standard','standard','standard','standard','standard','standard','standard','standard'},'SLDataType',{'SS_DOUBLE','SS_DOUBLE','SS_DOUBLE','SS_DOUBLE','SS_DOUBLE','SS_DOUBLE','SS_DOUBLE','SS_DOUBLE','SS_DOUBLE','SS_DOUBLE','SS_DOUBLE','SS_DOUBLE'},'DataType',{['signed int'],['unsigned int'],['signed int'],['unsigned int'],['unsigned int'],['unsigned int'],['unsigned int'],['signed int'],['unsigned int'],['unsigned int'],['unsigned int'],['signed int']},'ModeValue',{-1,-1,-1,-1,-1,-1,-1,-1,-1,-1,-1,-1}),'StatusSelected','no','TimeSelected','no','DeltaTimeSelected','no','BytePortSelected','no','MessageLengthSelected','no','TriggerPort',struct('Selected','no','TriggerType',0),'UserCoding',struct('Selected','no','InterfaceFile','UserDecodingFile','FcnName','UserDecodeFcn','InportSelected','no','InportWidth',1,'OutportSelected','no','OutportWidth',1),'EnablePortSelected','no','UseRXService','no','BoardType','DS1','BoardNo',2,'ControllerNo',2),'OFF',[]}},'TLCFileName',{{'rtican_rx_message','OFF',[]}})  RTISFcnParameters=struct('SFcnRTICANMessage','struct','TLCFileName','char')  RTIBlockParaDefault=struct('BoardTypeNo',4302,'BoardNo',1,'ChannelNo',1,'Parameters',struct('DataFileSupport',struct('DataFileSelectedMaster',0,'DataFileSelectedLocal',0,'DataFileName','','DataFileDate','','SelectedFile',['<no file selected>']),'Options',struct('StatusSelected',1,'TimeSelected',1,'DeltaTimeSelected',1,'BytePortSelected',0,'MessageLengthSelected',0,'TriggerPort',struct('Selected',0,'TriggerType','rising'),'UserCoding',struct('Selected',0,'InterfaceFile','UserDecodingFile','FcnName','UserDecodeFcn','InportSelected',0,'InportWidth',1,'OutportSelected',0,'OutportWidth',1),'EnablePortSelected',0,'SignalOnPortnameSelected',1,'UseRXService',0),'Message',struct('MsgOnBlocknameSelected',0,'MsgName',['RX Message'],'MsgIdFormat',0,'MsgId',100,'MsgLength',8,'NumSignals',1,'SampleTime',-1,'Signal',struct('SgnName',['RX signal'],'SgnStartBit',0,'SgnLength',8,'SgnType',0,'ModeValue',-1,'DataType',0,'SLDataType','SS_DOUBLE','ByteLayout',0,'Factor',1,'Offset',0,'Min',0,'Max',255,'SgnComment',{{}},'SgnUnit',''),'MsgIdNumFormat',0,'MsgComment',{{''}}),'Version',1.2,'general',struct('isFromLib',1)),'GroupId',struct('Group',{{'RTICAN'}},'No',1,'Behavior',{{'NAMECHANGE'}},'BlockType',{{'SINK'}},'NameChangeFlag',0),'SFcnRTICANMessage',struct('MsgType','RX','MsgName',['RX Message'],'MsgIdFormat','STD','MsgId',100,'MsgLength',8,'NumSignals',1,'SampleTime',-1,'Signal',struct('SgnName',['RX signal'],'SgnStartBit',0,'SgnLength',8,'SgnType','standard','ModeValue',-1,'DataType',['unsigned int'],'ByteLayout',['little endian'],'SLDataType','SS_DOUBLE','Factor',1,'Offset',0),'StatusSelected','yes','TimeSelected','yes','DeltaTimeSelected','yes','BytePortSelected','no','MessageLengthSelected','no','EnablePortSelected','no','UserCoding',struct('Selected','no','InterfaceFile','UserDecodingFile','FcnName','UserDecodeFcn','InportSelected','no','InportWidth',1,'OutportSelected','no','OutportWidth',1),'TriggerPort',struct('Selected','no','TriggerType','rising'),'UseRXService','no','BoardType','DS4302','BoardNo',1,'ControllerNo',1,'SFcnPortType','Scalar'),'TLCFileName','rtican_rx_message')
      settings: AttributesFormatString=Group Id: RTICAN4\n
  Out1 : Outport
  wires:
  Bus Creator/1 -> Out1/1  "Track02"
  ESR_Track02/1 -> Bus Creator/1  "CAN_TX_TRACK_RANGE_RATE_02"
  ESR_Track02/2 -> Bus Creator/2  "CAN_TX_TRACK_MED_RANGE_MODE_02"
  ESR_Track02/3 -> Bus Creator/3  "CAN_TX_TRACK_RANGE_ACCEL_02"
  ESR_Track02/4 -> Bus Creator/4  "CAN_TX_TRACK_WIDTH_02"
  ESR_Track02/5 -> Bus Creator/5  "CAN_TX_TRACK_ROLLING_COUNT_02"
  ESR_Track02/6 -> Bus Creator/6  "CAN_TX_TRACK_BRIDGE_OBJECT_02"
  ESR_Track02/7 -> Bus Creator/7  "CAN_TX_TRACK_RANGE_02"
  ESR_Track02/8 -> Bus Creator/8  "CAN_TX_TRACK_ANGLE_02"
  ESR_Track02/9 -> Bus Creator/9  "CAN_TX_TRACK_STATUS_02"
  ESR_Track02/10 -> Bus Creator/10  "CAN_TX_TRACK_ONCOMING_02"
  ESR_Track02/11 -> Bus Creator/11  "CAN_TX_TRACK_GROUPING_CHANGED_02"
  ESR_Track02/12 -> Bus Creator/12  "CAN_TX_TRACK_LAT_RATE_02"

== system Control_test/InputProcessing/RadarCanProcessing/Track03 ==
  Bus Creator : BusCreator  Inputs=12
  ESR_Track03 : rtican/RTICAN Receive (RX)   Reserved1=[]  Reserved2=[]  Reserved3=[]  Reserved4=[]  SfcnMessage=[]  Msg_Struct=[]  BoardTypeNo=[]  BoardNo=[]  ChannelNo=[]  Parameters=[]  DialogFcn=[]  UnitName=[]  Revision=[]  UnitValues=[]  DSProperties=struct('RTI',struct('Version',uint32(5),'BlockType',struct('isSLSource',uint8(1),'isSLSink',uint8(1),'isHWSource',uint8(0),'isHWSink',uint8(0),'isSetup',uint8(0),'isInline',uint8(1),'isNonInline',uint8(0),'isInterrupt',uint8(0),'isChannelwise',uint8(0)),'IOBoardType','RTICAN','UnitType','MESSAGE','Identifier','RX','DialogType','MSVC','BlockSet','RTICAN','SlaveProcessor','CAN'))  RTIBlockInterface=struct('OutputPortsWidth',int32([1 1 1 1 1 1 1 1 1 1 1 1]),'OutputPortsActive',[1 1 1 1 1 1 1 1 1 1 1 1],'OutputPortsName',{{'CAN_TX_TRACK_RANGE_RATE_03','CAN_TX_TRACK_MED_RANGE_MODE_03','CAN_TX_TRACK_RANGE_ACCEL_03','CAN_TX_TRACK_WIDTH_03','CAN_TX_TRACK_ROLLING_COUNT_03','CAN_TX_TRACK_BRIDGE_OBJECT_03','CAN_TX_TRACK_RANGE_03','CAN_TX_TRACK_ANGLE_03','CAN_TX_TRACK_STATUS_03','CAN_TX_TRACK_ONCOMING_03','CAN_TX_TRACK_GROUPING_CHANGED_03','CAN_TX_TRACK_LAT_RATE_03'}},'OutputPortsDataType',{{'SS_DOUBLE','SS_DOUBLE','SS_DOUBLE','SS_DOUBLE','SS_DOUBLE','SS_DOUBLE','SS_DOUBLE','SS_DOUBLE','SS_DOUBLE','SS_DOUBLE','SS_DOUBLE','SS_DOUBLE'}},'OutputPortsLabel',{{'CAN_TX_TRACK_RANGE_RATE_03','CAN_TX_TRACK_MED_RANGE_MODE_03','CAN_TX_TRACK_RANGE_ACCEL_03','CAN_TX_TRACK_WIDTH_03','CAN_TX_TRACK_ROLLING_COUNT_03','CAN_TX_TRACK_BRIDGE_OBJECT_03','CAN_TX_TRACK_RANGE_03','CAN_TX_TRACK_ANGLE_03','CAN_TX_TRACK_STATUS_03','CAN_TX_TRACK_ONCOMING_03','CAN_TX_TRACK_GROUPING_CHANGED_03','CAN_TX_TRACK_LAT_RATE_03'}},'OutputPortsLabelMode','ON','InputPortsWidth',int32(0),'InputPortsActive',0,'DialogFcn','rtican_message_interface_gui','BlockDisplay',{{'','center'}},'IconTransparency','on','ParameterTunableNames',{{}},'InitLevel',3,'BlockName',struct('Token',{{'ESR_Track03'}}),'SampleTime',{{0.01}},'TriggerPort',{{'none'}},'EnablePort',{{'none'}})  RTIBlockParameters=struct('BoardTypeNo',{{1,'OFF',[]}},'BoardNo',{{2,'ON',[1 16]}},'ChannelNo',{{2,'ON',[1 2]}},'Parameters',{{struct('DataFileSupport',struct('DataFileSelectedMaster',1,'DataFileSelectedLocal',1,'DataFileName','c:\users\mpc_car\documents\github\mpc-car\controller\dbcfiles\esr_dv3_64tgt.dbc|','DataFileDate',['26-Aug-2014 13:16:21'],'SelectedFile','..\..\dbcfiles\esr_dv3_64tgt.dbc','InterfaceFcn','rtican_dbc_file_parser'),'Options',struct('StatusSelected',0,'TimeSelected',0,'DeltaTimeSelected',0,'BytePortSelected',0,'MessageLengthSelected',0,'TriggerPort',struct('Selected',0,'TriggerType',0),'UserCoding',struct('Selected',0,'InterfaceFile','UserDecodingFile','FcnName','UserDecodeFcn','InportSelected',0,'InportWidth',1,'OutportSelected',0,'OutportWidth',1),'EnablePortSelected',0,'SignalOnPortnameSelected',1,'UseRXService',0),'Message',struct('MsgOnBlocknameSelected',1,'MsgName','ESR_Track03','MsgIdFormat',0,'MsgId',1282,'MsgLength',8,'NumSignals',12,'SampleTime',0.01,'Signal',struct('SgnName',{'CAN_TX_TRACK_RANGE_RATE_03','CAN_TX_TRACK_MED_RANGE_MODE_03','CAN_TX_TRACK_RANGE_ACCEL_03','CAN_TX_TRACK_WIDTH_03','CAN_TX_TRACK_ROLLING_COUNT_03','CAN_TX_TRACK_BRIDGE_OBJECT_03','CAN_TX_TRACK_RANGE_03','CAN_TX_TRACK_ANGLE_03','CAN_TX_TRACK_STATUS_03','CAN_TX_TRACK_ONCOMING_03','CAN_TX_TRACK_GROUPING_CHANGED_03','CAN_TX_TRACK_LAT_RATE_03'},'SgnStartBit',{0,14,16,26,30,31,32,43,53,56,57,58},'SgnLength',{14,2,10,4,1,1,11,10,3,1,1,6},'ByteLayout',{2,2,2,2,2,2,2,2,2,2,2,2},'Factor',{0.01,1,0.05,0.5,1,1,0.1,0.1,1,1,1,0.25},'Offset',{0,0,0,0,0,0,0,0,0,0,0,0},'SgnComment',{'','','','','','','','','','','',''},'SgnUnit',{'m/s','','m/s/s','m','','','m','deg','','','',''},'Min',{-81.92,0,-25.6,0,0,0,0,-51.2,0,0,0,-8},'Max',{81.91,3,25.55,7.5,1,0,204.7,51.1,7,0,0,7.75},'SgnType',{0,0,0,0,0,0,0,0,0,0,0,0},'SLDataType',{'SS_DOUBLE','SS_DOUBLE','SS_DOUBLE','SS_DOUBLE','SS_DOUBLE','SS_DOUBLE','SS_DOUBLE','SS_DOUBLE','SS_DOUBLE','SS_DOUBLE','SS_DOUBLE','SS_DOUBLE'},'DataType',{1,0,1,0,0,0,0,1,0,0,0,1},'ModeValue',{-1,-1,-1,-1,-1,-1,-1,-1,-1,-1,-1,-1}),'MsgIdNumFormat',0,'MsgComment',{{''}}),'Version',1.2,'general',struct('isFromLib',0)),'OFF',[]}},'GroupId',{{struct('Group',{{'RTICAN'}},'No',4,'Behavior',{{'NAMECHANGE'}},'BlockType',{{'SINK'}},'NameChangeFlag',0),'OFF',[]}},'SFcnRTICANMessage',{{struct('MsgType','RX','SFcnPortType','Scalar','MsgName','ESR_Track03','MsgIdFormat','STD','MsgId',1282,'MsgLength',8,'NumSignals',12,'SampleTime',0.01,'Signal',struct('SgnName',{'CAN_TX_TRACK_RANGE_RATE_03','CAN_TX_TRACK_MED_RANGE_MODE_03','CAN_TX_TRACK_RANGE_ACCEL_03','CAN_TX_TRACK_WIDTH_03','CAN_TX_TRACK_ROLLING_COUNT_03','CAN_TX_TRACK_BRIDGE_OBJECT_03','CAN_TX_TRACK_RANGE_03','CAN_TX_TRACK_ANGLE_03','CAN_TX_TRACK_STATUS_03','CAN_TX_TRACK_ONCOMING_03','CAN_TX_TRACK_GROUPING_CHANGED_03','CAN_TX_TRACK_LAT_RATE_03'},'SgnStartBit',{0,14,16,26,30,31,32,43,53,56,57,58},'SgnLength',{14,2,10,4,1,1,11,10,3,1,1,6},'ByteLayout',{['motorola back.'],['motorola back.'],['motorola back.'],['motorola back.'],['motorola back.'],['motorola back.'],['motorola back.'],['motorola back.'],['motorola back.'],['motorola back.'],['motorola back.'],['motorola back.']},'Factor',{0.01,1,0.05,0.5,1,1,0.1,0.1,1,1,1,0.25},'Offset',{0,0,0,0,0,0,0,0,0,0,0,0},'SgnType',{'standard','standard','standard','standard','standard','standard','standard','standard','standard','standard','standard','standard'},'SLDataType',{'SS_DOUBLE','SS_DOUBLE','SS_DOUBLE','SS_DOUBLE','SS_DOUBLE','SS_DOUBLE','SS_DOUBLE','SS_DOUBLE','SS_DOUBLE','SS_DOUBLE','SS_DOUBLE','SS_DOUBLE'},'DataType',{['signed int'],['unsigned int'],['signed int'],['unsigned int'],['unsigned int'],['unsigned int'],['unsigned int'],['signed int'],['unsigned int'],['unsigned int'],['unsigned int'],['signed int']},'ModeValue',{-1,-1,-1,-1,-1,-1,-1,-1,-1,-1,-1,-1}),'StatusSelected','no','TimeSelected','no','DeltaTimeSelected','no','BytePortSelected','no','MessageLengthSelected','no','TriggerPort',struct('Selected','no','TriggerType',0),'UserCoding',struct('Selected','no','InterfaceFile','UserDecodingFile','FcnName','UserDecodeFcn','InportSelected','no','InportWidth',1,'OutportSelected','no','OutportWidth',1),'EnablePortSelected','no','UseRXService','no','BoardType','DS1','BoardNo',2,'ControllerNo',2),'OFF',[]}},'TLCFileName',{{'rtican_rx_message','OFF',[]}})  RTISFcnParameters=struct('SFcnRTICANMessage','struct','TLCFileName','char')  RTIBlockParaDefault=struct('BoardTypeNo',4302,'BoardNo',1,'ChannelNo',1,'Parameters',struct('DataFileSupport',struct('DataFileSelectedMaster',0,'DataFileSelectedLocal',0,'DataFileName','','DataFileDate','','SelectedFile',['<no file selected>']),'Options',struct('StatusSelected',1,'TimeSelected',1,'DeltaTimeSelected',1,'BytePortSelected',0,'MessageLengthSelected',0,'TriggerPort',struct('Selected',0,'TriggerType','rising'),'UserCoding',struct('Selected',0,'InterfaceFile','UserDecodingFile','FcnName','UserDecodeFcn','InportSelected',0,'InportWidth',1,'OutportSelected',0,'OutportWidth',1),'EnablePortSelected',0,'SignalOnPortnameSelected',1,'UseRXService',0),'Message',struct('MsgOnBlocknameSelected',0,'MsgName',['RX Message'],'MsgIdFormat',0,'MsgId',100,'MsgLength',8,'NumSignals',1,'SampleTime',-1,'Signal',struct('SgnName',['RX signal'],'SgnStartBit',0,'SgnLength',8,'SgnType',0,'ModeValue',-1,'DataType',0,'SLDataType','SS_DOUBLE','ByteLayout',0,'Factor',1,'Offset',0,'Min',0,'Max',255,'SgnComment',{{}},'SgnUnit',''),'MsgIdNumFormat',0,'MsgComment',{{''}}),'Version',1.2,'general',struct('isFromLib',1)),'GroupId',struct('Group',{{'RTICAN'}},'No',1,'Behavior',{{'NAMECHANGE'}},'BlockType',{{'SINK'}},'NameChangeFlag',0),'SFcnRTICANMessage',struct('MsgType','RX','MsgName',['RX Message'],'MsgIdFormat','STD','MsgId',100,'MsgLength',8,'NumSignals',1,'SampleTime',-1,'Signal',struct('SgnName',['RX signal'],'SgnStartBit',0,'SgnLength',8,'SgnType','standard','ModeValue',-1,'DataType',['unsigned int'],'ByteLayout',['little endian'],'SLDataType','SS_DOUBLE','Factor',1,'Offset',0),'StatusSelected','yes','TimeSelected','yes','DeltaTimeSelected','yes','BytePortSelected','no','MessageLengthSelected','no','EnablePortSelected','no','UserCoding',struct('Selected','no','InterfaceFile','UserDecodingFile','FcnName','UserDecodeFcn','InportSelected','no','InportWidth',1,'OutportSelected','no','OutportWidth',1),'TriggerPort',struct('Selected','no','TriggerType','rising'),'UseRXService','no','BoardType','DS4302','BoardNo',1,'ControllerNo',1,'SFcnPortType','Scalar'),'TLCFileName','rtican_rx_message')
      settings: AttributesFormatString=Group Id: RTICAN4\n
  Out1 : Outport
  wires:
  Bus Creator/1 -> Out1/1  "Track03"
  ESR_Track03/1 -> Bus Creator/1  "CAN_TX_TRACK_RANGE_RATE_03"
  ESR_Track03/2 -> Bus Creator/2  "CAN_TX_TRACK_MED_RANGE_MODE_03"
  ESR_Track03/3 -> Bus Creator/3  "CAN_TX_TRACK_RANGE_ACCEL_03"
  ESR_Track03/4 -> Bus Creator/4  "CAN_TX_TRACK_WIDTH_03"
  ESR_Track03/5 -> Bus Creator/5  "CAN_TX_TRACK_ROLLING_COUNT_03"
  ESR_Track03/6 -> Bus Creator/6  "CAN_TX_TRACK_BRIDGE_OBJECT_03"
  ESR_Track03/7 -> Bus Creator/7  "CAN_TX_TRACK_RANGE_03"
  ESR_Track03/8 -> Bus Creator/8  "CAN_TX_TRACK_ANGLE_03"
  ESR_Track03/9 -> Bus Creator/9  "CAN_TX_TRACK_STATUS_03"
  ESR_Track03/10 -> Bus Creator/10  "CAN_TX_TRACK_ONCOMING_03"
  ESR_Track03/11 -> Bus Creator/11  "CAN_TX_TRACK_GROUPING_CHANGED_03"
  ESR_Track03/12 -> Bus Creator/12  "CAN_TX_TRACK_LAT_RATE_03"
